simulink model "ukol_9_model"  (R2017a)
settings: Solver=VariableStepAuto  StartTime=0.0  StopTime=30  MaxStep=1e-3  RelTol=1e-3  EnableMultiTasking=on
values from neighbouring files (symbols this model uses):
  A = [0 1; -1.44 -0.36]    [ukol_5_script.m]
  B = [0; 1]    [ukol_5_script.m]
  C_1 = [7.2 0]    [ukol_5_script.m]
  D = [0; 0]    [ukol_5_script.m]    (also in ukol_8_script.m = 0; ukol_9_script.m)
  k1 = 0.9821    [ukol_5_script.m]    (also in ukol_9_script.m = 0.982)
  k2 = 1.8188    [ukol_5_script.m]    (also in ukol_9_script.m)
  korekcni_zesileni = 1/chyba_zesileni    [ukol_5_script.m]
  L = [0.505555; 0.173555]    [ukol_8_script.m]
settings Model: Creator=kuhaj  LastModifiedBy=tomas
settings DataIOCC: LimitDataPoints=on
settings OptimizationCC: LifeSpan=inf
settings DebuggingCC: AllowSymbolicDim=off  SFUnexpectedBacktrackingDiag=warning  SFNoUnconditionalDefaultTransitionDiag=warning  SFExecutionAtInitializationDiag=none
settings ModelReferenceCC: PropagateSignalLabelsOutOfModel=off
settings GRTTargetCC: TargetLangStandard=C89/C90 (ANSI)
settings ConfigComp: CovMetricSettings=dw  CovHtmlReporting=on  CovSaveCumulativeToWorkspaceVar=on  CovSaveSingleToWorkspaceVar=on  CovExternalEMLEnable=off

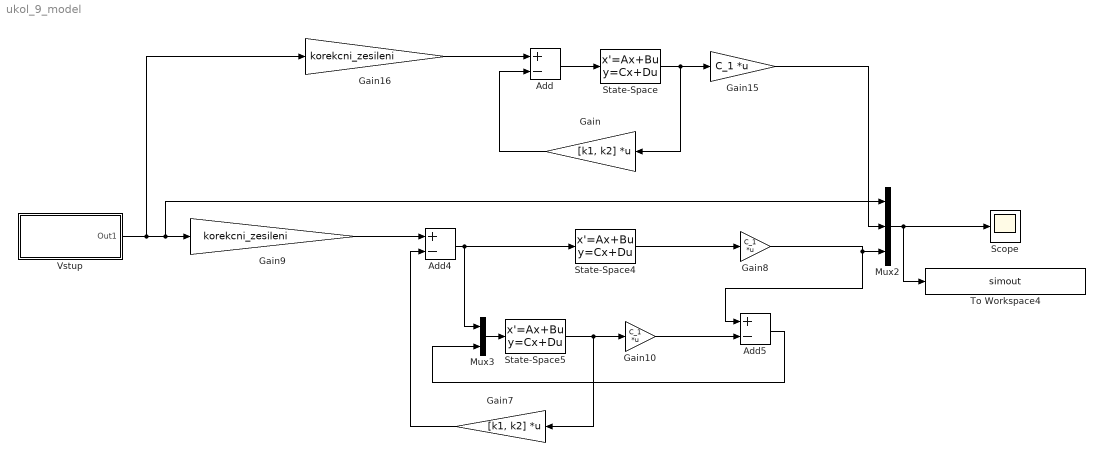
== system ukol_9_model ==
  Add : Sum  Inputs=+-
  Add4 : Sum  Inputs=+-
  Add5 : Sum  Inputs=+-
  Gain : Gain  Gain=[k1, k2]  Multiplication=Matrix(K*u)
  Gain10 : Gain  Gain=C_1  Multiplication=Matrix(K*u)
  Gain15 : Gain  Gain=C_1  Multiplication=Matrix(K*u)
  Gain16 : Gain  Gain=korekcni_zesileni
  Gain7 : Gain  Gain=[k1, k2]  Multiplication=Matrix(K*u)
  Gain8 : Gain  Gain=C_1  Multiplication=Matrix(K*u)
  Gain9 : Gain  Gain=korekcni_zesileni
  Mux2 : Mux  Inputs=3
  Mux3 : Mux  Inputs=2
  Scope : Scope
  State-Space : StateSpace  A=A  B=B  C=[1 0; 0 1]  D=D  X0=0
  State-Space4 : StateSpace  A=A  B=B  C=[1 0; 0 1]  D=D  X0=0
  State-Space5 : StateSpace  A=A  B=[B L]  C=[1 0; 0 1]  D=[0 0; 0 0]  X0=[0.3;-0.2]
  To Workspace4 : ToWorkspace  VariableName=simout  SaveFormat=Timeseries  SampleTime=-1
  Vstup : Subsystem
  wires:
  Gain7/1 -> Add4/2
  Add4/1 -> State-Space4/1, Mux3/1
  Gain9/1 -> Add4/1
  Mux2/1 -> To Workspace4/1, Scope/1
  Gain8/1 -> Add5/1, Mux2/3
  State-Space4/1 -> Gain8/1
  Mux3/1 -> State-Space5/1
  State-Space5/1 -> Gain10/1, Gain7/1
  Gain10/1 -> Add5/2
  Add5/1 -> Mux3/2
  Gain15/1 -> Mux2/2
  Vstup/1(Out1) -> Gain16/1, Mux2/1, Gain9/1
  Gain16/1 -> Add/1
  Gain/1 -> Add/2
  State-Space/1 -> Gain/1, Gain15/1
  Add/1 -> State-Space/1

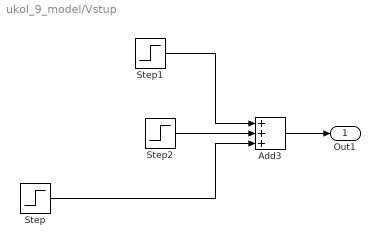
== system ukol_9_model/Vstup ==
  Add3 : Sum  Inputs=+++
  Step : Step  SampleTime=0
  Step1 : Step  Time=10  After=-4  SampleTime=0
  Step2 : Step  Time=20  After=8  SampleTime=0
  Out1 : Outport
  wires:
  Step/1 -> Add3/3
  Step1/1 -> Add3/1
  Step2/1 -> Add3/2
  Add3/1 -> Out1/1
